simulink model "SinglePhase_UPFC_Switching"  (R2024b)
settings: Solver=ode3  StartTime=0  StopTime=0.6  FixedStep=Ts_power  RelTol=1e-3
InitFcn:
  | f_grid = 50;
  | w0 = 2*pi*f_grid;
  | Vout_ref_rms = 220;
  | Vout_ref_pk = sqrt(2)*Vout_ref_rms;
  | Vgrid_pk = sqrt(2)*220;
  | Vgrid_sag_pk = sqrt(2)*176;
  | Vdc_ref = 400;
  | Cdc = 4700e-6;
  | Lsh = 4e-3;
  | Rsh = 0.35;
  | Lse = 1.5e-3;
  | Rse = 0.20;
  | Kpvdc = 0.45;
  | Kivdc = 8;
  | Kpq = 0.006;
  | Kiq = 0.35;
  | Kpi_sh = 12;
  | Kii_sh = 1200;
  | Kpv_se = 0.8;
  | Kiv_se = 120;
  | wc_v = 2*pi*40;
  | wc_q = 2*pi*25;
  | Qsh_ref_final = 500;
  | fsw = 10000;
  | Ts_power = 2e-6;
libraries: spsSeriesRLCBranchLib x8, spsGroundLib x6, spsVoltageMeasurementLib x4, spsCurrentMeasurementLib x3, spsRMSLib x2, spsUniversalBridgeLib x2, simulink x2, spsPLLLib x1, spsControlledVoltageSourceLib x1, spsLinearTransformerLib x1, spspowerguiLib x1
settings Model: Creator=17332  LastModifiedBy=26279
settings DataIOCC: SaveOutput=off  SignalLogging=off  SaveTime=off

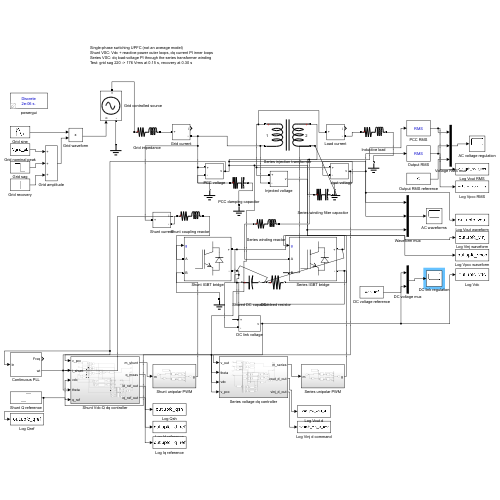
[thumbnail: Simulink's stored preview of the top-level diagram]
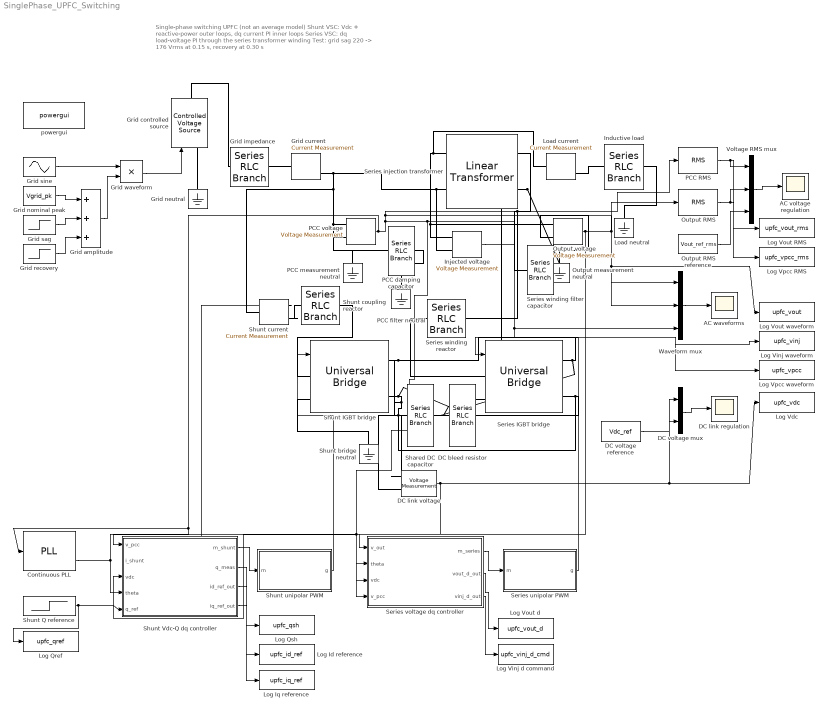
== system SinglePhase_UPFC_Switching ==
  note: Single-phase switching UPFC (not an average model)
      | Shunt VSC: Vdc + reactive-power outer loops, dq current PI inner loops
      | Series VSC: dq load-voltage PI through the series transformer winding
      | Test: grid sag 220 -> 176 Vrms at 0.15 s, recovery at 0.30 s
  AC voltage regulation : Scope
  AC waveforms : Scope
  Continuous PLL : spsPLLLib/PLL  Fmin=45  Par_Init=[0 50]  ParK=[180 3200 1]  TcD=1e-4  MaxRateChangeFreq=12  FilterCutOffFreq=25  Ts=0  AGC=on
  DC bleed resistor : spsSeriesRLCBranchLib/Series RLC Branch  LConnTagsString=__new0  RConnTagsString=__new0  BranchType=R  Resistance=20000  Inductance=1e-3  SetiL0=off  InitialCurrent=0  Capacitance=1e-6  Setx0=off  InitialVoltage=0  Measurements=None
  DC link regulation : Scope
  DC link voltage : spsVoltageMeasurementLib/Voltage Measurement  PhasorSimulation=off  OutputType=Complex  PSBequivalent=0
  DC voltage mux : Mux  Inputs=2
  DC voltage reference : Constant  Value=Vdc_ref
  Grid amplitude : Sum  Inputs=+++
  Grid controlled source : spsControlledVoltageSourceLib/Controlled Voltage Source  Initialize=on  Source_Type=AC  Amplitude=0  Phase=0  Frequency=0  Measurements=None
  Grid current : spsCurrentMeasurementLib/Current Measurement  PhasorSimulation=off  OutputType=Complex  PSBequivalent=0
  Grid impedance : spsSeriesRLCBranchLib/Series RLC Branch  LConnTagsString=__new0  RConnTagsString=__new0  BranchType=RL  Resistance=0.20  Inductance=2e-3  SetiL0=off  InitialCurrent=0  Capacitance=1e-6  Setx0=off  InitialVoltage=0  Measurements=None
  Grid neutral : spsGroundLib/Ground  LConnTagsString=a
  Grid nominal peak : Constant  Value=Vgrid_pk
  Grid recovery : Step  Time=0.30  After=Vgrid_pk-Vgrid_sag_pk  SampleTime=0
  Grid sag : Step  Time=0.15  After=Vgrid_sag_pk-Vgrid_pk  SampleTime=0
  Grid sine : Sin  Frequency=w0  SampleTime=0
  Grid waveform : Product
  Inductive load : spsSeriesRLCBranchLib/Series RLC Branch  LConnTagsString=__new0  RConnTagsString=__new0  BranchType=RL  Resistance=25  Inductance=10e-3  SetiL0=off  InitialCurrent=0  Capacitance=1e-6  Setx0=off  InitialVoltage=0  Measurements=None
  Injected voltage : spsVoltageMeasurementLib/Voltage Measurement  PhasorSimulation=off  OutputType=Complex  PSBequivalent=0
  Load current : spsCurrentMeasurementLib/Current Measurement  PhasorSimulation=off  OutputType=Complex  PSBequivalent=0
  Load neutral : spsGroundLib/Ground  LConnTagsString=a
  Log Id reference : ToWorkspace  VariableName=upfc_id_ref  SaveFormat=Structure With Time  SampleTime=-1
      settings: Decimation=10
  Log Iq reference : ToWorkspace  VariableName=upfc_iq_ref  SaveFormat=Structure With Time  SampleTime=-1
      settings: Decimation=10
  Log Qref : ToWorkspace  VariableName=upfc_qref  SaveFormat=Structure With Time  SampleTime=-1
      settings: Decimation=10
  Log Qsh : ToWorkspace  VariableName=upfc_qsh  SaveFormat=Structure With Time  SampleTime=-1
      settings: Decimation=10
  Log Vdc : ToWorkspace  VariableName=upfc_vdc  SaveFormat=Structure With Time  SampleTime=-1
      settings: Decimation=10
  Log Vinj d command : ToWorkspace  VariableName=upfc_vinj_d_cmd  SaveFormat=Structure With Time  SampleTime=-1
      settings: Decimation=10
  Log Vinj waveform : ToWorkspace  VariableName=upfc_vinj  SaveFormat=Structure With Time  SampleTime=-1
      settings: Decimation=10
  Log Vout RMS : ToWorkspace  VariableName=upfc_vout_rms  SaveFormat=Structure With Time  SampleTime=-1
      settings: Decimation=10
  Log Vout d : ToWorkspace  VariableName=upfc_vout_d  SaveFormat=Structure With Time  SampleTime=-1
      settings: Decimation=10
  Log Vout waveform : ToWorkspace  VariableName=upfc_vout  SaveFormat=Structure With Time  SampleTime=-1
      settings: Decimation=10
  Log Vpcc RMS : ToWorkspace  VariableName=upfc_vpcc_rms  SaveFormat=Structure With Time  SampleTime=-1
      settings: Decimation=10
  Log Vpcc waveform : ToWorkspace  VariableName=upfc_vpcc  SaveFormat=Structure With Time  SampleTime=-1
      settings: Decimation=10
  Output RMS : spsRMSLib/RMS  TrueRMS=on  Freq=50  RMSInit=220  Ts=0
  Output RMS reference : Constant  Value=Vout_ref_rms
  Output measurement neutral : spsGroundLib/Ground  LConnTagsString=a
  Output voltage : spsVoltageMeasurementLib/Voltage Measurement  PhasorSimulation=off  OutputType=Complex  PSBequivalent=0
  PCC RMS : spsRMSLib/RMS  TrueRMS=on  Freq=50  RMSInit=220  Ts=0
  PCC damping capacitor : spsSeriesRLCBranchLib/Series RLC Branch  LConnTagsString=__new0  RConnTagsString=__new0  BranchType=RC  Resistance=1  Inductance=1e-3  SetiL0=off  InitialCurrent=0  Capacitance=20e-6  Setx0=off  InitialVoltage=0  Measurements=None
  PCC filter neutral : spsGroundLib/Ground  LConnTagsString=a
  PCC measurement neutral : spsGroundLib/Ground  LConnTagsString=a
  PCC voltage : spsVoltageMeasurementLib/Voltage Measurement  PhasorSimulation=off  OutputType=Complex  PSBequivalent=0
  Series IGBT bridge : spsUniversalBridgeLib/Universal Bridge  Arms=2  SnubberResistance=1e5  SnubberCapacitance=inf  Device=IGBT / Diodes  Ron=1e-3  Lon=0  ForwardVoltages=[0.8 0.8]  ForwardVoltage=0  GTOparameters=[ 10e-6 , 20e-6 ]  IGBTparameters=[1e-6 2e-6]  Measurements=None  Measurements_2=None  converterType=Rectifier
  Series injection transformer : spsLinearTransformerLib/Linear Transformer  UNITS=pu  NominalPower=[5000 50]  winding1=[220 0.005 0.01]  winding2=[220 0.005 0.01]  ThreeWindings=off  winding3=[ 315e3 0.002 0.08 ]  RmLm=[500 500]  Measurements=None  DataType=off
  Series unipolar PWM : Subsystem
  Series voltage dq controller : Subsystem
  Series winding filter capacitor : spsSeriesRLCBranchLib/Series RLC Branch  LConnTagsString=__new0  RConnTagsString=__new0  BranchType=RC  Resistance=2  Inductance=1e-3  SetiL0=off  InitialCurrent=0  Capacitance=20e-6  Setx0=off  InitialVoltage=0  Measurements=None
  Series winding reactor : spsSeriesRLCBranchLib/Series RLC Branch  LConnTagsString=__new0  RConnTagsString=__new0  BranchType=RL  Resistance=Rse  Inductance=Lse  SetiL0=off  InitialCurrent=0  Capacitance=1e-6  Setx0=off  InitialVoltage=0  Measurements=None
  Shared DC capacitor : spsSeriesRLCBranchLib/Series RLC Branch  LConnTagsString=__new0  RConnTagsString=__new0  BranchType=C  Resistance=1  Inductance=1e-3  SetiL0=off  InitialCurrent=0  Capacitance=Cdc  Setx0=on  InitialVoltage=Vdc_ref  Measurements=None
  Shunt IGBT bridge : spsUniversalBridgeLib/Universal Bridge  Arms=2  SnubberResistance=1e5  SnubberCapacitance=inf  Device=IGBT / Diodes  Ron=1e-3  Lon=0  ForwardVoltages=[0.8 0.8]  ForwardVoltage=0  GTOparameters=[ 10e-6 , 20e-6 ]  IGBTparameters=[1e-6 2e-6]  Measurements=None  Measurements_2=None  converterType=Rectifier
  Shunt Q reference : Step  Time=0.22  After=Qsh_ref_final  SampleTime=0
  Shunt Vdc-Q dq controller : Subsystem
  Shunt bridge neutral : spsGroundLib/Ground  LConnTagsString=a
  Shunt coupling reactor : spsSeriesRLCBranchLib/Series RLC Branch  LConnTagsString=__new0  RConnTagsString=__new0  BranchType=RL  Resistance=Rsh  Inductance=Lsh  SetiL0=off  InitialCurrent=0  Capacitance=1e-6  Setx0=off  InitialVoltage=0  Measurements=None
  Shunt current : spsCurrentMeasurementLib/Current Measurement  PhasorSimulation=off  OutputType=Complex  PSBequivalent=0
  Shunt unipolar PWM : Subsystem
  Voltage RMS mux : Mux  Inputs=3
  Waveform mux : Mux  Inputs=3
  powergui : spspowerguiLib/powergui  Priority=1  SimulationMode=Discrete  SampleTime=Ts_power  frequency=60  Iterations=50  frequencyindice=0  Pbase=100e6  ErrMax=1e-4  UnitsV=kV  UnitsW=MW  buscounter=0  FunctionMessages=off  echomessages=off  EnableUseOfTLC=off  CurrentSourceSwitches=off  DisableSnubberDevices=off  DisableRonSwitches=off  DisableVfSwitches=off  DisplayEquations=off  AutomaticDiscreteSolvers=off  SolverType=Tustin/Backward Euler (TBE)  Interpol=off  ExternalGateDelay=off  methode=off  Ts=100  x0status=blocks  SPID=on  SwTol=0  HookPort=off  NonlinearTolerance=1e-4  nMaxIteration=100  ContinueOnMaxIteration=off  RestoreLinks=warning  ResistiveCurrentMeasurement=off  Frange=[0:2:500]  Ylog=off  Xlog=on  ShowGrid=off  save=off  variable=ZData  structure=0  ZoomFFT=off  StartTime=0.0  cycles=1  DisplayStyle=1  fundamental=60  FreqAxis=off  MaxFrequency=1000  frequencyindicesteady=1  RmsSteady=1  display=off
  wires:
  Grid sine/1 -> Grid waveform/1
  Grid nominal peak/1 -> Grid amplitude/1
  Grid sag/1 -> Grid amplitude/2
  Grid recovery/1 -> Grid amplitude/3
  Grid amplitude/1 -> Grid waveform/2
  Grid waveform/1 -> Grid controlled source/1
  PCC voltage/1 -> Series voltage dq controller/4(v_pcc), Log Vpcc waveform/1, PCC RMS/1, Waveform mux/1, Continuous PLL/1, Shunt Vdc-Q dq controller/1(v_pcc)
  Shunt current/1 -> Shunt Vdc-Q dq controller/2(i_shunt)
  DC link voltage/1 -> Shunt Vdc-Q dq controller/3(vdc), Series voltage dq controller/3(vdc), DC voltage mux/1, Log Vdc/1
  Continuous PLL/2 -> Shunt Vdc-Q dq controller/4(theta), Series voltage dq controller/2(theta)
  Shunt Q reference/1 -> Shunt Vdc-Q dq controller/5(q_ref), Log Qref/1
  Shunt Vdc-Q dq controller/1(m_shunt) -> Shunt unipolar PWM/1(m)
  Shunt unipolar PWM/1(g) -> Shunt IGBT bridge/1
  Output voltage/1 -> Waveform mux/2, Log Vout waveform/1, Output RMS/1, Series voltage dq controller/1(v_out)
  Series voltage dq controller/1(m_series) -> Series unipolar PWM/1(m)
  Series unipolar PWM/1(g) -> Series IGBT bridge/1
  PCC RMS/1 -> Voltage RMS mux/1, Log Vpcc RMS/1
  Output RMS/1 -> Voltage RMS mux/2, Log Vout RMS/1
  Output RMS reference/1 -> Voltage RMS mux/3
  Voltage RMS mux/1 -> AC voltage regulation/1
  DC voltage reference/1 -> DC voltage mux/2
  DC voltage mux/1 -> DC link regulation/1
  Injected voltage/1 -> Waveform mux/3, Log Vinj waveform/1
  Waveform mux/1 -> AC waveforms/1
  Shunt Vdc-Q dq controller/2(q_meas) -> Log Qsh/1
  Series voltage dq controller/2(vout_d_out) -> Log Vout d/1
  Series voltage dq controller/3(vinj_d_out) -> Log Vinj d command/1
  Shunt Vdc-Q dq controller/3(id_ref_out) -> Log Id reference/1
  Shunt Vdc-Q dq controller/4(iq_ref_out) -> Log Iq reference/1
  connections:
  Grid controlled source/LConn1 -- Grid neutral/LConn1
  Grid controlled source/RConn1 -- Grid impedance/LConn1
  Grid impedance/RConn1 -- Grid current/LConn1
  Grid current/RConn1 -- PCC voltage/LConn1 -- PCC damping capacitor/LConn1 -- Shunt current/LConn1 -- Injected voltage/LConn2 -- Series injection transformer/LConn2
  Load current/LConn1 -- Output voltage/LConn1 -- Injected voltage/LConn1 -- Series injection transformer/LConn1
  Load current/RConn1 -- Inductive load/LConn1
  Inductive load/RConn1 -- Load neutral/LConn1
  PCC voltage/LConn2 -- PCC measurement neutral/LConn1
  PCC damping capacitor/RConn1 -- PCC filter neutral/LConn1
  Output voltage/LConn2 -- Output measurement neutral/LConn1
  Shunt current/RConn1 -- Shunt coupling reactor/LConn1
  Shunt coupling reactor/RConn1 -- Shunt IGBT bridge/LConn1
  Shunt IGBT bridge/LConn2 -- Shunt bridge neutral/LConn1
  Series IGBT bridge/LConn1 -- Series winding reactor/LConn1
  Series winding reactor/RConn1 -- Series injection transformer/RConn1 -- Series winding filter capacitor/LConn1
  Series injection transformer/RConn2 -- Series IGBT bridge/LConn2 -- Series winding filter capacitor/RConn1
  Shunt IGBT bridge/RConn1 -- Series IGBT bridge/RConn1 -- DC bleed resistor/LConn1 -- Shared DC capacitor/LConn1 -- DC link voltage/LConn1
  Shunt IGBT bridge/RConn2 -- DC link voltage/LConn2 -- Series IGBT bridge/RConn2 -- DC bleed resistor/RConn1 -- Shared DC capacitor/RConn1

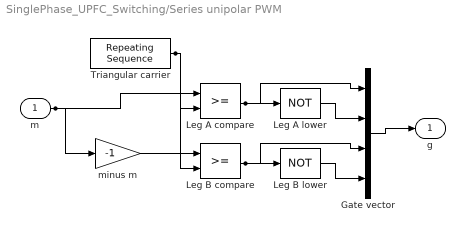
== system SinglePhase_UPFC_Switching/Series unipolar PWM ==
  m : Inport
  Gate vector : Mux
  Leg A compare : RelationalOperator  OutDataTypeStr=boolean  RndMeth=Simplest  InputSameDT=off
  Leg A lower : Logic  Operator=NOT  AllPortsSameDT=off  OutDataTypeStr=boolean
  Leg B compare : RelationalOperator  OutDataTypeStr=boolean  RndMeth=Simplest  InputSameDT=off
  Leg B lower : Logic  Operator=NOT  AllPortsSameDT=off  OutDataTypeStr=boolean
  Triangular carrier : simulink/Sources/Repeating Sequence  rep_seq_t=[0 0.5 1]/fsw  rep_seq_y=[-1 1 -1]
  minus m : Gain  Gain=-1
  g : Outport
  wires:
  m/1 -> Leg A compare/1, minus m/1
  minus m/1 -> Leg B compare/1
  Triangular carrier/1 -> Leg A compare/2, Leg B compare/2
  Leg A compare/1 -> Leg A lower/1, Gate vector/1
  Leg B compare/1 -> Leg B lower/1, Gate vector/3
  Leg A lower/1 -> Gate vector/2
  Leg B lower/1 -> Gate vector/4
  Gate vector/1 -> g/1

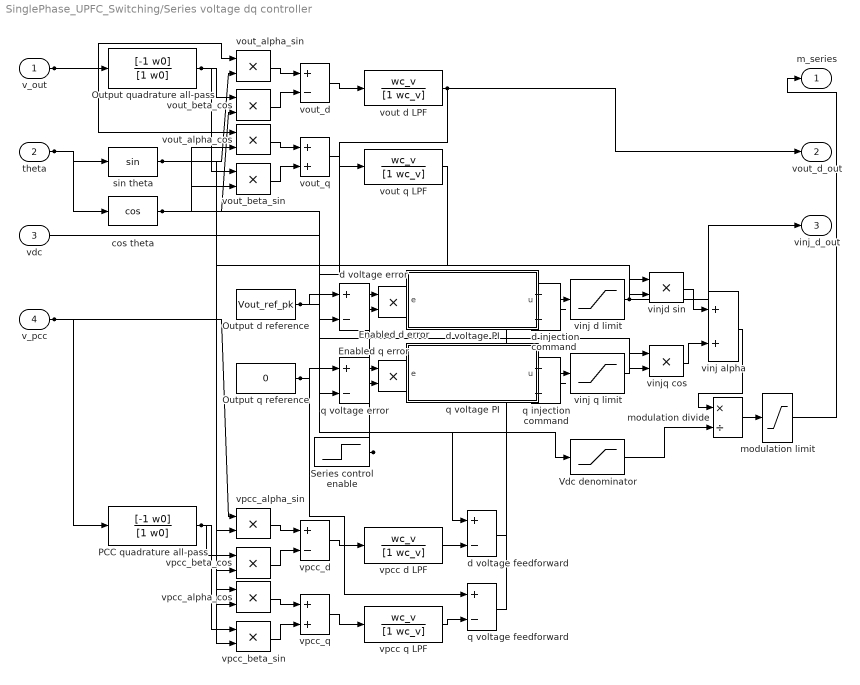
== system SinglePhase_UPFC_Switching/Series voltage dq controller ==
  v_out : Inport
  theta : Inport  Port=2
  vdc : Inport  Port=3
  v_pcc : Inport  Port=4
  Enabled d error : Product
  Enabled q error : Product
  Output d reference : Constant  Value=Vout_ref_pk
  Output q reference : Constant  Value=0
  Output quadrature all-pass : TransferFcn  Numerator=[-1 w0]  Denominator=[1 w0]
  PCC quadrature all-pass : TransferFcn  Numerator=[-1 w0]  Denominator=[1 w0]
  Series control enable : Step  Time=0.06  SampleTime=0
  Vdc denominator : Saturate  UpperLimit=inf  LowerLimit=100
  cos theta : Trigonometry  Operator=cos
  d injection command : Sum
  d voltage PI : Subsystem
  d voltage error : Sum  Inputs=+-
  d voltage feedforward : Sum  Inputs=+-
  modulation divide : Product  Inputs=*/
  modulation limit : Saturate  UpperLimit=0.95  LowerLimit=-0.95
  q injection command : Sum
  q voltage PI : Subsystem
  q voltage error : Sum  Inputs=+-
  q voltage feedforward : Sum  Inputs=+-
  sin theta : Trigonometry
  vinj alpha : Sum
  vinj d limit : Saturate  UpperLimit=100  LowerLimit=-100
  vinj q limit : Saturate  UpperLimit=100  LowerLimit=-100
  vinjd sin : Product
  vinjq cos : Product
  vout d LPF : TransferFcn  Numerator=wc_v  Denominator=[1 wc_v]
  vout q LPF : TransferFcn  Numerator=wc_v  Denominator=[1 wc_v]
  vout_alpha_cos : Product
  vout_alpha_sin : Product
  vout_beta_cos : Product
  vout_beta_sin : Product
  vout_d : Sum  Inputs=+-
  vout_q : Sum
  vpcc d LPF : TransferFcn  Numerator=wc_v  Denominator=[1 wc_v]
  vpcc q LPF : TransferFcn  Numerator=wc_v  Denominator=[1 wc_v]
  vpcc_alpha_cos : Product
  vpcc_alpha_sin : Product
  vpcc_beta_cos : Product
  vpcc_beta_sin : Product
  vpcc_d : Sum  Inputs=+-
  vpcc_q : Sum
  m_series : Outport
  vout_d_out : Outport  Port=2
  vinj_d_out : Outport  Port=3
  wires:
  v_out/1 -> vout_alpha_sin/1, vout_alpha_cos/1, Output quadrature all-pass/1
  sin theta/1 -> vout_alpha_sin/2, vout_beta_sin/2, vpcc_alpha_sin/2, vpcc_beta_sin/2, vinjd sin/2
  Output quadrature all-pass/1 -> vout_beta_cos/1, vout_beta_sin/1
  cos theta/1 -> vout_beta_cos/2, vout_alpha_cos/2, vpcc_beta_cos/2, vpcc_alpha_cos/2, vinjq cos/2
  vout_alpha_sin/1 -> vout_d/1
  vout_beta_cos/1 -> vout_d/2
  vout_alpha_cos/1 -> vout_q/1
  vout_beta_sin/1 -> vout_q/2
  theta/1 -> sin theta/1, cos theta/1
  vout_d/1 -> vout d LPF/1
  vout_q/1 -> vout q LPF/1
  vout d LPF/1 -> vout_d_out/1, d voltage error/2
  v_pcc/1 -> vpcc_alpha_sin/1, vpcc_alpha_cos/1, PCC quadrature all-pass/1
  PCC quadrature all-pass/1 -> vpcc_beta_cos/1, vpcc_beta_sin/1
  vpcc_alpha_sin/1 -> vpcc_d/1
  vpcc_beta_cos/1 -> vpcc_d/2
  vpcc_alpha_cos/1 -> vpcc_q/1
  vpcc_beta_sin/1 -> vpcc_q/2
  vpcc_d/1 -> vpcc d LPF/1
  vpcc_q/1 -> vpcc q LPF/1
  Output d reference/1 -> d voltage error/1, d voltage feedforward/1
  Output q reference/1 -> q voltage error/1, q voltage feedforward/1
  vout q LPF/1 -> q voltage error/2
  d voltage error/1 -> Enabled d error/1
  q voltage error/1 -> Enabled q error/1
  Series control enable/1 -> Enabled d error/2, Enabled q error/2
  Enabled d error/1 -> d voltage PI/1(e)
  Enabled q error/1 -> q voltage PI/1(e)
  vpcc d LPF/1 -> d voltage feedforward/2
  vpcc q LPF/1 -> q voltage feedforward/2
  d voltage PI/1(u) -> d injection command/1
  d voltage feedforward/1 -> d injection command/2
  q voltage PI/1(u) -> q injection command/1
  q voltage feedforward/1 -> q injection command/2
  d injection command/1 -> vinj d limit/1
  q injection command/1 -> vinj q limit/1
  vinj d limit/1 -> vinj_d_out/1, vinjd sin/1
  vinj q limit/1 -> vinjq cos/1
  vinjd sin/1 -> vinj alpha/1
  vinjq cos/1 -> vinj alpha/2
  vdc/1 -> Vdc denominator/1
  vinj alpha/1 -> modulation divide/1
  Vdc denominator/1 -> modulation divide/2
  modulation divide/1 -> modulation limit/1
  modulation limit/1 -> m_series/1

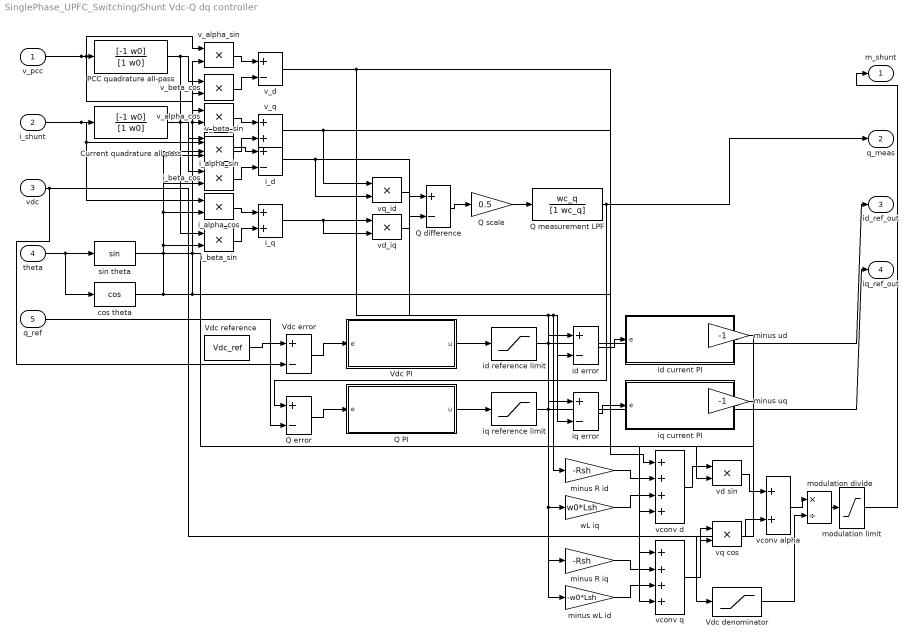
== system SinglePhase_UPFC_Switching/Shunt Vdc-Q dq controller ==
  v_pcc : Inport
  i_shunt : Inport  Port=2
  vdc : Inport  Port=3
  theta : Inport  Port=4
  q_ref : Inport  Port=5
  Current quadrature all-pass : TransferFcn  Numerator=[-1 w0]  Denominator=[1 w0]
  PCC quadrature all-pass : TransferFcn  Numerator=[-1 w0]  Denominator=[1 w0]
  Q PI : Subsystem
  Q difference : Sum  Inputs=+-
  Q error : Sum  Inputs=+-
  Q measurement LPF : TransferFcn  Numerator=wc_q  Denominator=[1 wc_q]
  Q scale : Gain  Gain=0.5
  Vdc PI : Subsystem
  Vdc denominator : Saturate  UpperLimit=inf  LowerLimit=100
  Vdc error : Sum  Inputs=+-
  Vdc reference : Constant  Value=Vdc_ref
  cos theta : Trigonometry  Operator=cos
  i_alpha_cos : Product
  i_alpha_sin : Product
  i_beta_cos : Product
  i_beta_sin : Product
  i_d : Sum  Inputs=+-
  i_q : Sum
  id current PI : Subsystem
  id error : Sum  Inputs=+-
  id reference limit : Saturate  UpperLimit=12  LowerLimit=-12
  iq current PI : Subsystem
  iq error : Sum  Inputs=+-
  iq reference limit : Saturate  UpperLimit=8  LowerLimit=-8
  minus R id : Gain  Gain=-Rsh
  minus R iq : Gain  Gain=-Rsh
  minus ud : Gain  Gain=-1
  minus uq : Gain  Gain=-1
  minus wL id : Gain  Gain=-w0*Lsh
  modulation divide : Product  Inputs=*/
  modulation limit : Saturate  UpperLimit=0.95  LowerLimit=-0.95
  sin theta : Trigonometry
  v_alpha_cos : Product
  v_alpha_sin : Product
  v_beta_cos : Product
  v_beta_sin : Product
  v_d : Sum  Inputs=+-
  v_q : Sum
  vconv alpha : Sum
  vconv d : Sum  Inputs=++++
  vconv q : Sum  Inputs=++++
  vd sin : Product
  vd_iq : Product
  vq cos : Product
  vq_id : Product
  wL iq : Gain  Gain=w0*Lsh
  m_shunt : Outport
  q_meas : Outport  Port=2
  id_ref_out : Outport  Port=3
  iq_ref_out : Outport  Port=4
  wires:
  v_pcc/1 -> v_alpha_sin/1, v_alpha_cos/1, PCC quadrature all-pass/1
  sin theta/1 -> v_alpha_sin/2, vd sin/2, v_beta_sin/2, i_alpha_sin/2, i_beta_sin/2
  PCC quadrature all-pass/1 -> v_beta_cos/1, v_beta_sin/1
  cos theta/1 -> v_beta_cos/2, v_alpha_cos/2, vq cos/2, i_beta_cos/2, i_alpha_cos/2
  v_alpha_sin/1 -> v_d/1
  v_beta_cos/1 -> v_d/2
  v_alpha_cos/1 -> v_q/1
  v_beta_sin/1 -> v_q/2
  i_shunt/1 -> i_alpha_sin/1, i_alpha_cos/1, Current quadrature all-pass/1
  Current quadrature all-pass/1 -> i_beta_cos/1, i_beta_sin/1
  i_alpha_sin/1 -> i_d/1
  i_beta_cos/1 -> i_d/2
  i_alpha_cos/1 -> i_q/1
  i_beta_sin/1 -> i_q/2
  theta/1 -> sin theta/1, cos theta/1
  v_q/1 -> vq_id/1, vconv q/1
  i_d/1 -> id error/2, minus R id/1, minus wL id/1, vq_id/2
  v_d/1 -> vd_iq/1, vconv d/1
  i_q/1 -> wL iq/1, minus R iq/1, iq error/2, vd_iq/2
  vq_id/1 -> Q difference/1
  vd_iq/1 -> Q difference/2
  Q difference/1 -> Q scale/1
  Q scale/1 -> Q measurement LPF/1
  Q measurement LPF/1 -> q_meas/1, Q error/1
  Vdc reference/1 -> Vdc error/1
  vdc/1 -> Vdc error/2, Vdc denominator/1
  Vdc error/1 -> Vdc PI/1(e)
  Vdc PI/1(u) -> id reference limit/1
  id reference limit/1 -> id_ref_out/1, id error/1
  q_ref/1 -> Q error/2
  Q error/1 -> Q PI/1(e)
  Q PI/1(u) -> iq reference limit/1
  iq reference limit/1 -> iq_ref_out/1, iq error/1
  id error/1 -> id current PI/1(e)
  iq error/1 -> iq current PI/1(e)
  minus R id/1 -> vconv d/2
  wL iq/1 -> vconv d/3
  id current PI/1(u) -> minus ud/1
  minus ud/1 -> vconv d/4
  minus R iq/1 -> vconv q/2
  minus wL id/1 -> vconv q/3
  iq current PI/1(u) -> minus uq/1
  minus uq/1 -> vconv q/4
  vconv d/1 -> vd sin/1
  vconv q/1 -> vq cos/1
  vd sin/1 -> vconv alpha/1
  vq cos/1 -> vconv alpha/2
  vconv alpha/1 -> modulation divide/1
  Vdc denominator/1 -> modulation divide/2
  modulation divide/1 -> modulation limit/1
  modulation limit/1 -> m_shunt/1

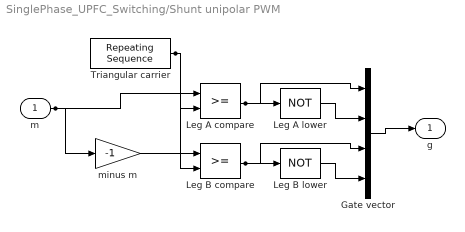
== system SinglePhase_UPFC_Switching/Shunt unipolar PWM ==
  m : Inport
  Gate vector : Mux
  Leg A compare : RelationalOperator  OutDataTypeStr=boolean  RndMeth=Simplest  InputSameDT=off
  Leg A lower : Logic  Operator=NOT  AllPortsSameDT=off  OutDataTypeStr=boolean
  Leg B compare : RelationalOperator  OutDataTypeStr=boolean  RndMeth=Simplest  InputSameDT=off
  Leg B lower : Logic  Operator=NOT  AllPortsSameDT=off  OutDataTypeStr=boolean
  Triangular carrier : simulink/Sources/Repeating Sequence  rep_seq_t=[0 0.5 1]/fsw  rep_seq_y=[-1 1 -1]
  minus m : Gain  Gain=-1
  g : Outport
  wires:
  m/1 -> Leg A compare/1, minus m/1
  minus m/1 -> Leg B compare/1
  Triangular carrier/1 -> Leg A compare/2, Leg B compare/2
  Leg A compare/1 -> Leg A lower/1, Gate vector/1
  Leg B compare/1 -> Leg B lower/1, Gate vector/3
  Leg A lower/1 -> Gate vector/2
  Leg B lower/1 -> Gate vector/4
  Gate vector/1 -> g/1

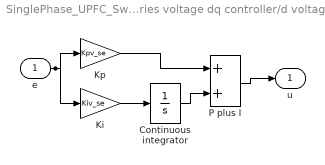
== system SinglePhase_UPFC_Switching/Series voltage dq controller/d voltage PI ==
  e : Inport
  Continuous integrator : Integrator
  Ki : Gain  Gain=Kiv_se
  Kp : Gain  Gain=Kpv_se
  P plus I : Sum
  u : Outport
  wires:
  e/1 -> Kp/1, Ki/1
  Ki/1 -> Continuous integrator/1
  Kp/1 -> P plus I/1
  Continuous integrator/1 -> P plus I/2
  P plus I/1 -> u/1

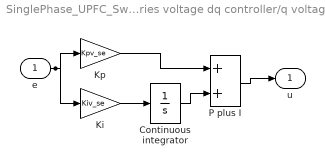
== system SinglePhase_UPFC_Switching/Series voltage dq controller/q voltage PI ==
  e : Inport
  Continuous integrator : Integrator
  Ki : Gain  Gain=Kiv_se
  Kp : Gain  Gain=Kpv_se
  P plus I : Sum
  u : Outport
  wires:
  e/1 -> Kp/1, Ki/1
  Ki/1 -> Continuous integrator/1
  Kp/1 -> P plus I/1
  Continuous integrator/1 -> P plus I/2
  P plus I/1 -> u/1

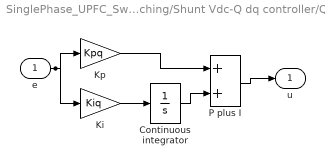
== system SinglePhase_UPFC_Switching/Shunt Vdc-Q dq controller/Q PI ==
  e : Inport
  Continuous integrator : Integrator
  Ki : Gain  Gain=Kiq
  Kp : Gain  Gain=Kpq
  P plus I : Sum
  u : Outport
  wires:
  e/1 -> Kp/1, Ki/1
  Ki/1 -> Continuous integrator/1
  Kp/1 -> P plus I/1
  Continuous integrator/1 -> P plus I/2
  P plus I/1 -> u/1

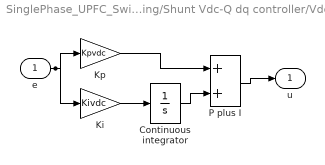
== system SinglePhase_UPFC_Switching/Shunt Vdc-Q dq controller/Vdc PI ==
  e : Inport
  Continuous integrator : Integrator
  Ki : Gain  Gain=Kivdc
  Kp : Gain  Gain=Kpvdc
  P plus I : Sum
  u : Outport
  wires:
  e/1 -> Kp/1, Ki/1
  Ki/1 -> Continuous integrator/1
  Kp/1 -> P plus I/1
  Continuous integrator/1 -> P plus I/2
  P plus I/1 -> u/1

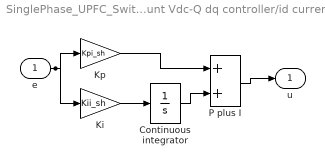
== system SinglePhase_UPFC_Switching/Shunt Vdc-Q dq controller/id current PI ==
  e : Inport
  Continuous integrator : Integrator
  Ki : Gain  Gain=Kii_sh
  Kp : Gain  Gain=Kpi_sh
  P plus I : Sum
  u : Outport
  wires:
  e/1 -> Kp/1, Ki/1
  Ki/1 -> Continuous integrator/1
  Kp/1 -> P plus I/1
  Continuous integrator/1 -> P plus I/2
  P plus I/1 -> u/1

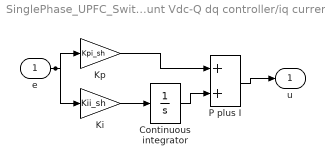
== system SinglePhase_UPFC_Switching/Shunt Vdc-Q dq controller/iq current PI ==
  e : Inport
  Continuous integrator : Integrator
  Ki : Gain  Gain=Kii_sh
  Kp : Gain  Gain=Kpi_sh
  P plus I : Sum
  u : Outport
  wires:
  e/1 -> Kp/1, Ki/1
  Ki/1 -> Continuous integrator/1
  Kp/1 -> P plus I/1
  Continuous integrator/1 -> P plus I/2
  P plus I/1 -> u/1
